simulink model "LIM_MO_Pso"  (R2016a)
settings: Solver=ode45  StartTime=0.0  StopTime=5
InitFcn:
  | %LIM in d-q referance
  | 
  |       Rs = 1.25;
  |       Rr = 2.7;
  |       Ls = 40.1e-3;
  |       Lr = 33.1e-3;
  |       Lm = 32.6e-3;
  |       tau =  0.0641;
  |       p = 4;
  |       D = 0.286;
  |       m = 8;
  |       ff=0;
  |      Tr=Lr/Rr;
  |     segma = 1-(Lm^2)/(Ls*Lr);
  |     sigma= segma;
  |        R=[Rs 0 0 0;0 Rs 0 0;0 0 Rr 0;0 0 0 Rr];
  |    R1=Rr*[1 0 1 0;0 0 0 0;1 0 1 0;0 0 0 0];%f(q)
  |    L=[Ls 0 0 0;0 Ls+Lm 0 Lm;0 0 Lr 0;0 Lm 0 Lr];
  |    L1=Lm*[1 0 1 0;0 0 0 0;1 0 1 0;0 0 0 0];%(1-f(q))
  |    M1=[0 -Ls-Lm 0 -Lm;Ls 0 0 0;0 0 0 0;0 0 0 0];
  |    M11=Lm*[0 0 0 0;1 0 1 0;0 0 0 0;0 0 0 0] ; %(1-f(q))
  |    M2=[0 0 0 0;0 0 0 0;0 -Lm 0 -Lr;0 0 Lr 0];
  |    M22=Lm*[0 0 0 0;0 0 0 0;0 0 0 0;1 0 1 0];%1-f(q)
  | 
  | 
  | Kpw = 7.8184
  | Kiw  = 55
  | Kpf = 6.9181
  | Kif = 996.637
  | Kpd = 8.9732
  | Kid  = 6792.1647
  | Kpq = 8.0997
  | Kiq = 6387.3475
StopFcn:
  |  figure(1)
  | plot(t,w,'LineWidth',2)
  | xlabel ('Time (s)','FontWeight','bold','FontSize',12)
  | ylabel ('speed (m/s)','FontWeight','bold','FontSize',12)
  | grid
  | 
  | 
  | figure(2)
  | plot(t,FF,'LineWidth',2)
  | xlabel ('Time (s)','FontWeight','bold','FontSize',12)
  | ylabel ('Thrust force (N)','FontWeight','bold','FontSize',12)
  | grid
  | 
  | 
  | figure(3)
  | plot(t,ids,'LineWidth',2)
  | xlabel ('Time (s)','FontWeight','bold','FontSize',12)
  | ylabel ('ids (A)','FontWeight','bold','FontSize',12)
  | grid
  | 
  | 
  | figure(4)
  | plot(t,iqs,'LineWidth',2)
  | xlabel ('Time (s)','FontWeight','bold','FontSize',12)
  | ylabel ('iqs (A)','FontWeight','bold','FontSize',12)
  | grid
  | 
  | figure(5)
  | plot(t,phdr,'LineWidth',2)
  | xlabel ('Time (s)','FontWeight','bold','FontSize',12)
  | ylabel ('phdr (Wb)','FontWeight','bold','FontSize',12)
  | grid
  | 
  | figure(6)
  | plot(t,phqr,'LineWidth',2)
  | xlabel ('Time (s)','FontWeight','bold','FontSize',12)
  | ylabel ('phqr (Wb)','FontWeight','bold','FontSize',12)
  | grid
libraries: simulink_need_slupdate x2, simulink x2
settings Model: Creator=DaLLaL  LastModifiedBy=DaLLaL
settings DebuggingCC: MaxConsecutiveZCsMsg=none

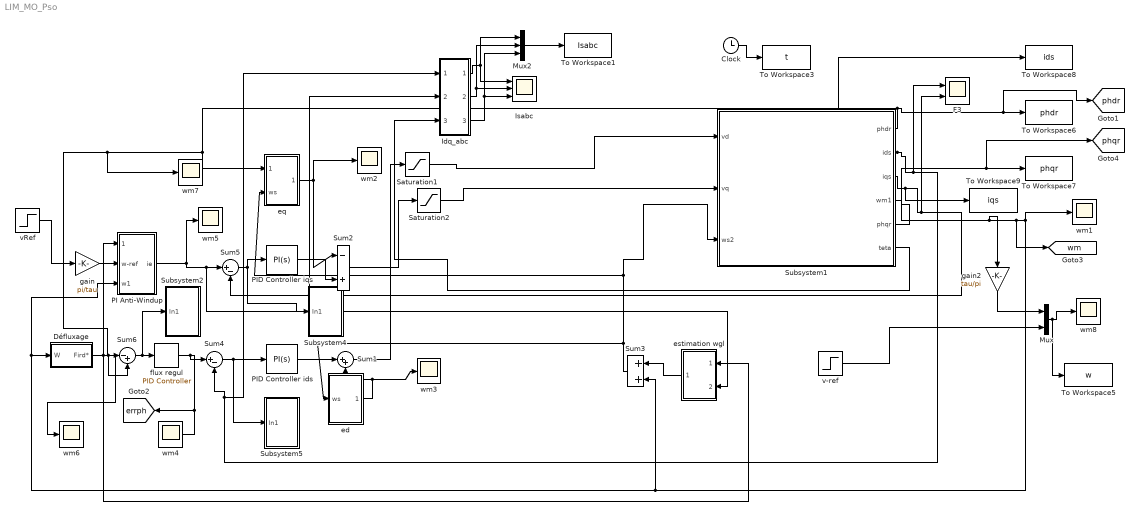
== system LIM_MO_Pso ==
  Clock : Clock
  Défluxage : Subsystem  mask{fref=0.4, Wn=300}
      mask prompts: fref "flux reference"; Wn "vitesse nominale"
  F3 : Scope  NumInputPorts=2
  Idq_abc : Subsystem
  Isabc : Scope  NumInputPorts=3
  Mux : Mux  Inputs=2
  Mux2 : Mux  Inputs=3
  PI Anti-Windup : Subsystem
  PID Controller ids : simulink/Continuous/PID Controller  Controller=PI  TimeDomain=Continuous-time  SampleTime=-1  IntegratorMethod=Forward Euler  FilterMethod=Forward Euler  Form=Parallel  UseFilter=on  ControllerParametersSource=internal  P=Kpd  I=Kid  D=0  N=100  InitialConditionSource=internal  InitialConditionForIntegrator=0  InitialConditionForFilter=0  ExternalReset=none  LimitOutput=off  UpperSaturationLimit=inf  LowerSaturationLimit=-inf  LinearizeAsGain=off  AntiWindupMode=none  Kb=1  TrackingMode=off  Kt=1  PParamMin=[]  PParamMax=[]  IParamMin=[]  IParamMax=[]  DParamMin=[]  DParamMax=[]  NParamMin=[]  NParamMax=[]  KbParamMin=[]  KbParamMax=[]  KtParamMin=[]  KtParamMax=[]  POutMin=[]  POutMax=[]  IOutMin=[]  IOutMax=[]  DOutMin=[]  DOutMax=[]  NOutMin=[]  NOutMax=[]  KbOutMin=[]  KbOutMax=[]  KtOutMin=[]  KtOutMax=[]  IntegratorOutMin=[]  IntegratorOutMax=[]  FilterOutMin=[]  FilterOutMax=[]  SumOutMin=[]  SumOutMax=[]  SumI1OutMin=[]  SumI1OutMax=[]  SumI2OutMin=[]  SumI2OutMax=[]  SumI3OutMin=[]  SumI3OutMax=[]  SumDOutMin=[]  SumDOutMax=[]  SaturationOutMin=[]  SaturationOutMax=[]  IntegratorContinuousStateAttributes=''  IntegratorStateMustResolveToSignalObject=off  IntegratorRTWStateStorageClass=Auto  FilterContinuousStateAttributes=''  FilterStateMustResolveToSignalObject=off  FilterRTWStateStorageClass=Auto  DifferentiatorICPrevScaledInput=0  DifferentiatorOutMin=[]  DifferentiatorOutMax=[]
  PID Controller iqs : simulink/Continuous/PID Controller  Controller=PI  TimeDomain=Continuous-time  SampleTime=-1  IntegratorMethod=Forward Euler  FilterMethod=Forward Euler  Form=Parallel  UseFilter=on  ControllerParametersSource=internal  P=Kpq  I=Kiq  D=0  N=100  InitialConditionSource=internal  InitialConditionForIntegrator=0  InitialConditionForFilter=0  ExternalReset=none  LimitOutput=off  UpperSaturationLimit=inf  LowerSaturationLimit=-inf  LinearizeAsGain=off  AntiWindupMode=none  Kb=1  TrackingMode=off  Kt=1  PParamMin=[]  PParamMax=[]  IParamMin=[]  IParamMax=[]  DParamMin=[]  DParamMax=[]  NParamMin=[]  NParamMax=[]  KbParamMin=[]  KbParamMax=[]  KtParamMin=[]  KtParamMax=[]  POutMin=[]  POutMax=[]  IOutMin=[]  IOutMax=[]  DOutMin=[]  DOutMax=[]  NOutMin=[]  NOutMax=[]  KbOutMin=[]  KbOutMax=[]  KtOutMin=[]  KtOutMax=[]  IntegratorOutMin=[]  IntegratorOutMax=[]  FilterOutMin=[]  FilterOutMax=[]  SumOutMin=[]  SumOutMax=[]  SumI1OutMin=[]  SumI1OutMax=[]  SumI2OutMin=[]  SumI2OutMax=[]  SumI3OutMin=[]  SumI3OutMax=[]  SumDOutMin=[]  SumDOutMax=[]  SaturationOutMin=[]  SaturationOutMax=[]  IntegratorContinuousStateAttributes=''  IntegratorStateMustResolveToSignalObject=off  IntegratorRTWStateStorageClass=Auto  FilterContinuousStateAttributes=''  FilterStateMustResolveToSignalObject=off  FilterRTWStateStorageClass=Auto  DifferentiatorICPrevScaledInput=0  DifferentiatorOutMin=[]  DifferentiatorOutMax=[]
  Saturation1 : Saturate  UpperLimit=600  LowerLimit=-600
  Saturation2 : Saturate  UpperLimit=600  LowerLimit=-600
  Subsystem1 : Subsystem
  Subsystem2 : Subsystem
  Subsystem4 : Subsystem
  Subsystem5 : Subsystem
  Sum1 : Sum  Inputs=|++
  Sum2 : Sum  Inputs=|-+
  Sum3 : Sum  Inputs=|++
  Sum4 : Sum  Inputs=|+-
  Sum5 : Sum  Inputs=|+-
  Sum6 : Sum  Inputs=|-+
  To Workspace1 : ToWorkspace  VariableName=Isabc  SampleTime=-1
  To Workspace3 : ToWorkspace  VariableName=t  SampleTime=-1
  To Workspace5 : ToWorkspace  VariableName=w  SampleTime=-1
  To Workspace6 : ToWorkspace  VariableName=phdr  SampleTime=-1
  To Workspace7 : ToWorkspace  VariableName=phqr  SampleTime=-1
  To Workspace8 : ToWorkspace  VariableName=ids  SampleTime=-1
  To Workspace9 : ToWorkspace  VariableName=iqs  SampleTime=-1
  ed : Subsystem
  eq : Subsystem
  estimation wgl : Subsystem
  flux regul : simulink_need_slupdate/PID Controller  P=Kpf  I=Kif  D=0
  gain : Gain  Gain=pi/tau
  gain2 : Gain  Gain=tau/pi
  v-ref : Step  Time=4  Before=3  After=4  SampleTime=0
  vRef : Step  Time=4  Before=3  After=4  SampleTime=0
  wm{1..8} (8 alike) : Scope
  tag scope: errph=global, phdr=global, phqr=global, wm=global
  wires:
  Subsystem1/2(ids) -> F3/1, Idq_abc/1(Vd), Sum4/2, To Workspace8/1
  Sum4/1 -> Subsystem5/1(In1), PID Controller ids/1
  Subsystem1/3(iqs) -> F3/2, Sum5/2, Idq_abc/2(Vq), To Workspace9/1
  Subsystem1/1(phdr) -> [phdr], To Workspace6/1, eq/1(phdr), Sum6/1, wm7/1
  PID Controller ids/1 -> Sum1/1
  eq/1(eqs) -> Sum2/1, wm2/1
  PI Anti-Windup/1(ie) -> Sum5/1, estimation wgl/2(iqsref), wm5/1
  Sum5/1 -> Subsystem4/1(In1), PID Controller iqs/1
  flux regul/1 -> Sum4/1, wm4/1, [errph]
  Défluxage/1(Fird*) -> wm6/1, Sum6/2, estimation wgl/1(phdr), PI Anti-Windup/1(phder)
  Sum3/1 -> Subsystem1/3(ws2), eq/2(ws), ed/1(ws)
  PID Controller iqs/1 -> Sum2/2
  Sum6/1 -> Subsystem2/1(In1), flux regul/1
  Subsystem1/5(phqr) -> [phqr], To Workspace7/1
  Mux/1 -> wm8/1, To Workspace5/1
  estimation wgl/1(wgl) -> Sum3/1
  Subsystem1/4(wm1) -> gain2/1, [wm], wm1/1, PI Anti-Windup/3(w1), Défluxage/1(W), Sum3/2
  Clock/1 -> To Workspace3/1
  ed/1(eds) -> Sum1/2, wm3/1
  Subsystem1/6(teta) -> Idq_abc/3(teta)
  Sum2/1 -> Saturation2/1
  Sum1/1 -> Saturation1/1
  vRef/1 -> gain/1
  gain/1 -> PI Anti-Windup/2(w-ref)
  v-ref/1 -> Mux/2
  Idq_abc/3(Vc) -> Mux2/3, Isabc/3
  Idq_abc/2(Vb) -> Mux2/2, Isabc/2
  Idq_abc/1(Va) -> Mux2/1, Isabc/1
  Mux2/1 -> To Workspace1/1
  gain2/1 -> Mux/1
  Saturation1/1 -> Subsystem1/1(vd)
  Saturation2/1 -> Subsystem1/2(vq)

== system LIM_MO_Pso/Défluxage ==
  W : Inport
  defluxage : Subsystem  mask(Defluxage){Phiref=1, Wn=Wn}
      mask prompts: Phiref "Phiref :"; Wn "Wn :"
      mask help: Defluxage
  Fird* : Outport
  wires:
  defluxage/1(fref) -> Fird*/1
  W/1 -> defluxage/1(w)

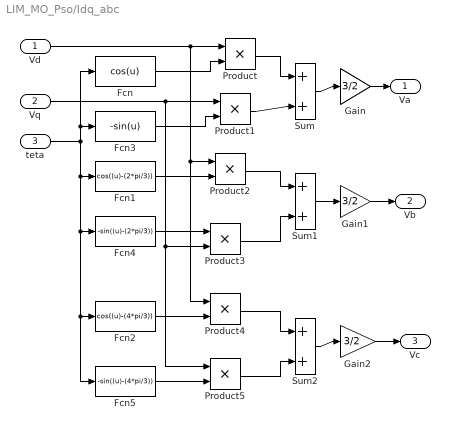
== system LIM_MO_Pso/Idq_abc ==
  Vd : Inport
  Vq : Inport  Port=2
  teta : Inport  Port=3
  Fcn : Fcn  Expr=cos(u)
  Fcn1 : Fcn  Expr=cos((u)-(2*pi/3))
  Fcn2 : Fcn  Expr=cos((u)-(4*pi/3))
  Fcn3 : Fcn  Expr=-sin(u)
  Fcn4 : Fcn  Expr=-sin((u)-(2*pi/3))
  Fcn5 : Fcn  Expr=-sin((u)-(4*pi/3))
  Gain : Gain  Gain=3/2  SaturateOnIntegerOverflow=on  OutDataTypeStr=Inherit: Same as input  ParamDataTypeStr=Inherit: Same as input
  Gain1 : Gain  Gain=3/2  SaturateOnIntegerOverflow=on  OutDataTypeStr=Inherit: Same as input  ParamDataTypeStr=Inherit: Same as input
  Gain2 : Gain  Gain=3/2  SaturateOnIntegerOverflow=on  OutDataTypeStr=Inherit: Same as input  ParamDataTypeStr=Inherit: Same as input
  Product{,1..5} (6 alike) : Product  SaturateOnIntegerOverflow=on  InputSameDT=on  OutDataTypeStr=Inherit: Same as first input
  Sum : Sum  Inputs=|++  SaturateOnIntegerOverflow=on  InputSameDT=on  OutDataTypeStr=Inherit: Same as first input
  Sum1 : Sum  Inputs=|++  SaturateOnIntegerOverflow=on  InputSameDT=on  OutDataTypeStr=Inherit: Same as first input
  Sum2 : Sum  Inputs=|++  SaturateOnIntegerOverflow=on  InputSameDT=on  OutDataTypeStr=Inherit: Same as first input
  Va : Outport
  Vb : Outport  Port=2
  Vc : Outport  Port=3
  wires:
  Gain2/1 -> Vc/1
  Gain1/1 -> Vb/1
  Gain/1 -> Va/1
  Sum2/1 -> Gain2/1
  Sum1/1 -> Gain1/1
  Sum/1 -> Gain/1
  Product5/1 -> Sum2/2
  Product4/1 -> Sum2/1
  Product3/1 -> Sum1/2
  Product2/1 -> Sum1/1
  Product1/1 -> Sum/2
  Product/1 -> Sum/1
  teta/1 -> Fcn5/1, Fcn2/1, Fcn4/1, Fcn1/1, Fcn3/1, Fcn/1
  Fcn5/1 -> Product5/2
  Fcn2/1 -> Product4/2
  Fcn4/1 -> Product3/1
  Fcn1/1 -> Product2/2
  Vq/1 -> Product5/1, Product3/2, Product1/1
  Vd/1 -> Product4/1, Product2/1, Product/1
  Fcn3/1 -> Product1/2
  Fcn/1 -> Product/2

== system LIM_MO_Pso/PI Anti-Windup ==
  phder : Inport
  w-ref : Inport  Port=2
  w1 : Inport  Port=3
  PID Controller2 : simulink_need_slupdate/PID Controller  P=Kpw  I=Kiw  D=0
  Subsystem : Subsystem
  Subsystem2 : Subsystem
  Sum : Sum  Inputs=|+-  SaturateOnIntegerOverflow=on
  ie : Outport
  wires:
  Sum/1 -> PID Controller2/1
  PID Controller2/1 -> Subsystem2/1(In1), Subsystem/2(ce*)
  phder/1 -> Subsystem/1(phder)
  w1/1 -> Sum/2
  w-ref/1 -> Sum/1
  Subsystem/1(ie*) -> ie/1

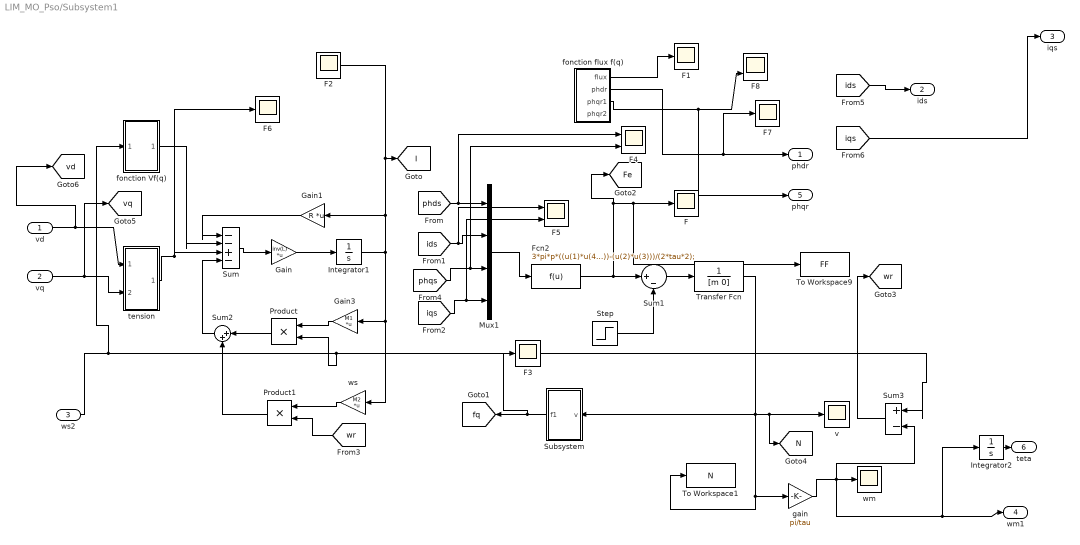
== system LIM_MO_Pso/Subsystem1 ==
  vd : Inport
  vq : Inport  Port=2
  ws2 : Inport  Port=3
  F{,1..3,6..7} (6 alike) : Scope
  F4 : Scope  NumInputPorts=2
  F5 : Scope  NumInputPorts=2
  F8 : Scope  NumInputPorts=2
  Fcn2 : Fcn  Expr=3*pi*p*((u(1)*u(4))-(u(2)*u(3)))/(2*tau*2);
  Gain : Gain  Gain=inv(L)  Multiplication=Matrix(K*u)
  Gain1 : Gain  Gain=R  Multiplication=Matrix(K*u)
  Gain3 : Gain  Gain=M1  Multiplication=Matrix(K*u)
  Integrator1 : Integrator
  Integrator2 : Integrator
  Mux1 : Mux
  Product : Product  RndMeth=Zero
  Product1 : Product  RndMeth=Zero
  Step : Step  After=50  SampleTime=0
  Subsystem : Subsystem
  Sum : Sum  Inputs=|--+-
  Sum1 : Sum  Inputs=|+-
  Sum2 : Sum  Inputs=|++
  Sum3 : Sum  Inputs=|+-
  To Workspace1 : ToWorkspace  VariableName=N  SampleTime=-1
  To Workspace9 : ToWorkspace  VariableName=FF  SampleTime=-1
  Transfer Fcn : TransferFcn  Denominator=[m 0]
  fonction Vf(q) : Subsystem
  fonction flux f(q) : Subsystem
  gain : Gain  Gain=pi/tau
  tension : Subsystem
  v : Scope
  wm : Scope
  ws : Gain  Gain=M2  Multiplication=Matrix(K*u)
  phdr : Outport
  ids : Outport  Port=2
  iqs : Outport  Port=3
  wm1 : Outport  Port=4
  phqr : Outport  Port=5
  teta : Outport  Port=6
  tag scope: Fe=global, I=global, N=global, fq=global, vd=global, vq=global, wr=global
  wires:
  Gain/1 -> Integrator1/1
  Integrator1/1 -> Gain3/1, ws/1, Gain1/1, [I], F2/1
  Gain3/1 -> Product/1
  Sum/1 -> Gain/1
  ws/1 -> Product1/1
  Product1/1 -> Sum2/2
  Product/1 -> Sum2/1
  [wr] -> Product1/2
  Gain1/1 -> Sum/1
  Sum2/1 -> Sum/4
  Subsystem/1(f1) -> [fq], F3/1
  fonction Vf(q)/1(Out1) -> Sum/2
  Fcn2/1 -> [Fe], F/1, To Workspace9/1, Sum1/1
  Step/1 -> Sum1/2
  Sum1/1 -> Transfer Fcn/1
  Transfer Fcn/1 -> To Workspace1/1, gain/1, [N], v/1, Subsystem/1(v)
  gain/1 -> wm/1, Sum3/2, wm1/1, Integrator2/1
  Sum3/1 -> [wr]
  [phds] -> Mux1/1, F4/1
  [ids] -> Mux1/2, F5/1
  [iqs] -> Mux1/4, F5/2
  [phqs] -> Mux1/3, F4/2
  Mux1/1 -> Fcn2/1
  fonction flux f(q)/1(flux) -> F1/1
  fonction flux f(q)/2(phdr) -> phdr/1, F7/1
  [ids] -> ids/1
  [iqs] -> iqs/1
  tension/1(V (v)) -> Sum/3, F6/1
  ws2/1 -> Product/2, Sum3/1, fonction Vf(q)/1(ws2)
  vd/1 -> [vd], tension/1(In2)
  vq/1 -> [vq], tension/2(In1)
  fonction flux f(q)/3(phqr1) -> F8/2, phqr/1
  Integrator2/1 -> teta/1

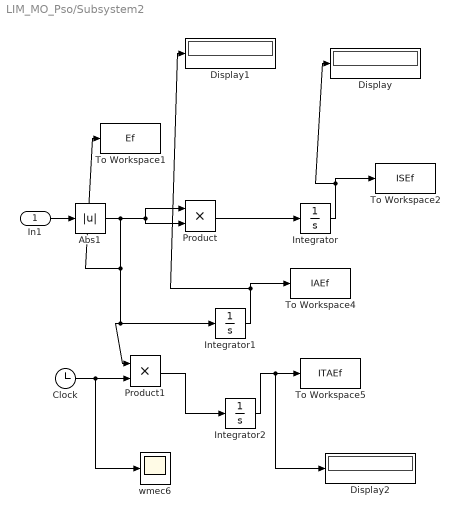
== system LIM_MO_Pso/Subsystem2 ==
  In1 : Inport
  Abs1 : Abs
  Clock : Clock
      settings: Decimation=4
  Display : Display
  Display1 : Display
  Display2 : Display
  Integrator : Integrator
  Integrator1 : Integrator
  Integrator2 : Integrator
  Product : Product  RndMeth=Zero
  Product1 : Product  RndMeth=Zero
  To Workspace1 : ToWorkspace  VariableName=Ef  SampleTime=-1
      settings: MaxDataPoints=1
  To Workspace2 : ToWorkspace  VariableName=ISEf  SampleTime=-1
      settings: MaxDataPoints=1
  To Workspace4 : ToWorkspace  VariableName=IAEf  SampleTime=-1
      settings: MaxDataPoints=1
  To Workspace5 : ToWorkspace  VariableName=ITAEf  SampleTime=-1
      settings: MaxDataPoints=1
  wmec6 : Scope
  wires:
  In1/1 -> Abs1/1
  Product1/1 -> Integrator2/1
  Integrator2/1 -> Display2/1, To Workspace5/1
  Clock/1 -> Product1/2, wmec6/1
  Integrator1/1 -> Display1/1, To Workspace4/1
  Abs1/1 -> Product/1, Product/2, Product1/1, Integrator1/1, To Workspace1/1
  Integrator/1 -> Display/1, To Workspace2/1
  Product/1 -> Integrator/1

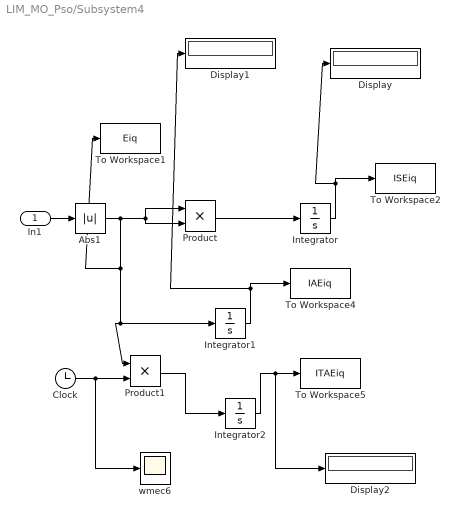
== system LIM_MO_Pso/Subsystem4 ==
  In1 : Inport
  Abs1 : Abs
  Clock : Clock
      settings: Decimation=4
  Display : Display
  Display1 : Display
  Display2 : Display
  Integrator : Integrator
  Integrator1 : Integrator
  Integrator2 : Integrator
  Product : Product  RndMeth=Zero
  Product1 : Product  RndMeth=Zero
  To Workspace1 : ToWorkspace  VariableName=Eiq  SampleTime=-1
      settings: MaxDataPoints=1
  To Workspace2 : ToWorkspace  VariableName=ISEiq  SampleTime=-1
      settings: MaxDataPoints=1
  To Workspace4 : ToWorkspace  VariableName=IAEiq  SampleTime=-1
      settings: MaxDataPoints=1
  To Workspace5 : ToWorkspace  VariableName=ITAEiq  SampleTime=-1
      settings: MaxDataPoints=1
  wmec6 : Scope
  wires:
  Product/1 -> Integrator/1
  Integrator/1 -> To Workspace2/1, Display/1
  Abs1/1 -> To Workspace1/1, Integrator1/1, Product1/1, Product/2, Product/1
  Integrator1/1 -> To Workspace4/1, Display1/1
  Clock/1 -> wmec6/1, Product1/2
  Integrator2/1 -> To Workspace5/1, Display2/1
  Product1/1 -> Integrator2/1
  In1/1 -> Abs1/1

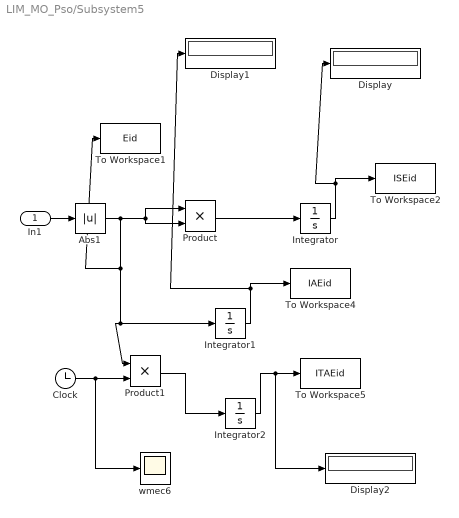
== system LIM_MO_Pso/Subsystem5 ==
  In1 : Inport
  Abs1 : Abs
  Clock : Clock
      settings: Decimation=4
  Display : Display
  Display1 : Display
  Display2 : Display
  Integrator : Integrator
  Integrator1 : Integrator
  Integrator2 : Integrator
  Product : Product  RndMeth=Zero
  Product1 : Product  RndMeth=Zero
  To Workspace1 : ToWorkspace  VariableName=Eid  SampleTime=-1
      settings: MaxDataPoints=1
  To Workspace2 : ToWorkspace  VariableName=ISEid  SampleTime=-1
      settings: MaxDataPoints=1
  To Workspace4 : ToWorkspace  VariableName=IAEid  SampleTime=-1
      settings: MaxDataPoints=1
  To Workspace5 : ToWorkspace  VariableName=ITAEid  SampleTime=-1
      settings: MaxDataPoints=1
  wmec6 : Scope
  wires:
  In1/1 -> Abs1/1
  Product1/1 -> Integrator2/1
  Integrator2/1 -> Display2/1, To Workspace5/1
  Clock/1 -> Product1/2, wmec6/1
  Integrator1/1 -> Display1/1, To Workspace4/1
  Abs1/1 -> Product/1, Product/2, Product1/1, Integrator1/1, To Workspace1/1
  Integrator/1 -> Display/1, To Workspace2/1
  Product/1 -> Integrator/1

== system LIM_MO_Pso/ed ==
  ws : Inport
  Gain2 : Gain  Gain=(Ls+Lm)-(Lm*Lm/(Lm+Lr))
  Product2 : Product  RndMeth=Zero
  eds : Outport
  wires:
  ws/1 -> Gain2/1
  [iqs] -> Product2/1
  Gain2/1 -> Product2/2
  Product2/1 -> eds/1

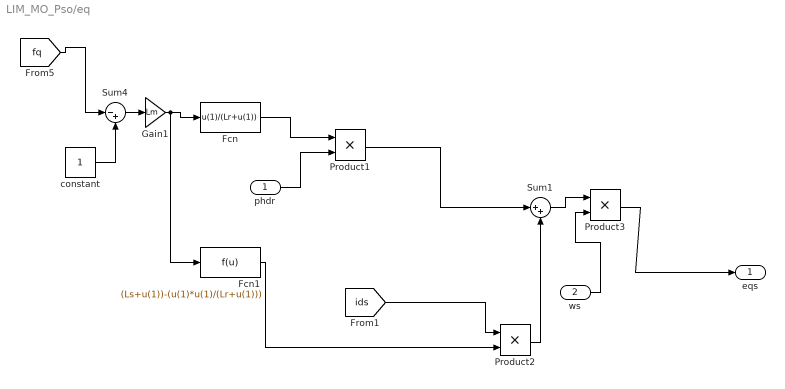
== system LIM_MO_Pso/eq ==
  phdr : Inport
  ws : Inport  Port=2
  Fcn : Fcn  Expr=u(1)/(Lr+u(1))
  Fcn1 : Fcn  Expr=(Ls+u(1))-(u(1)*u(1)/(Lr+u(1)))
  Gain1 : Gain  Gain=Lm
  Product1 : Product  RndMeth=Zero
  Product2 : Product  RndMeth=Zero
  Product3 : Product  RndMeth=Zero
  Sum1 : Sum  Inputs=|++
  Sum4 : Sum  Inputs=|-+
  constant : Constant
  eqs : Outport
  wires:
  [fq] -> Sum4/1
  constant/1 -> Sum4/2
  Sum4/1 -> Gain1/1
  [ids] -> Product2/1
  Fcn1/1 -> Product2/2
  phdr/1 -> Product1/2
  Fcn/1 -> Product1/1
  Gain1/1 -> Fcn/1, Fcn1/1
  Product1/1 -> Sum1/1
  Product2/1 -> Sum1/2
  Sum1/1 -> Product3/1
  ws/1 -> Product3/2
  Product3/1 -> eqs/1

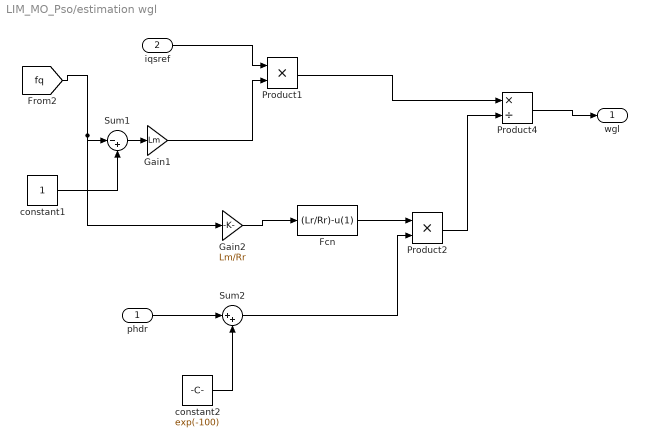
== system LIM_MO_Pso/estimation wgl ==
  phdr : Inport
  iqsref : Inport  Port=2
  Fcn : Fcn  Expr=(Lr/Rr)-u(1)
  Gain1 : Gain  Gain=Lm
  Gain2 : Gain  Gain=Lm/Rr
  Product1 : Product  RndMeth=Zero
  Product2 : Product  RndMeth=Zero
  Product4 : Product  Inputs=*/  RndMeth=Zero
  Sum1 : Sum  Inputs=|-+
  Sum2 : Sum  Inputs=|++
  constant1 : Constant
  constant2 : Constant  Value=exp(-100)
  wgl : Outport
  wires:
  phdr/1 -> Sum2/1
  constant2/1 -> Sum2/2
  iqsref/1 -> Product1/1
  Product4/1 -> wgl/1
  [fq] -> Sum1/1, Gain2/1
  constant1/1 -> Sum1/2
  Sum1/1 -> Gain1/1
  Gain1/1 -> Product1/2
  Gain2/1 -> Fcn/1
  Fcn/1 -> Product2/1
  Sum2/1 -> Product2/2
  Product2/1 -> Product4/2
  Product1/1 -> Product4/1

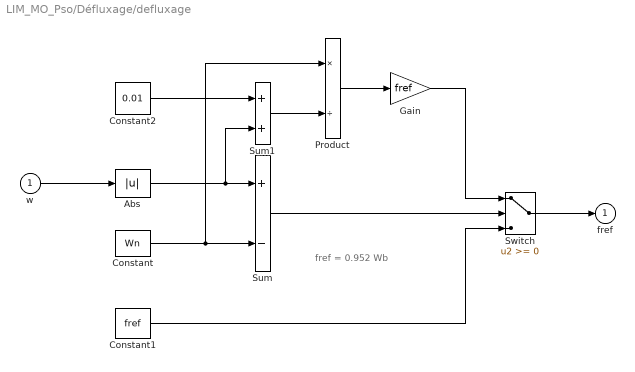
== system LIM_MO_Pso/Défluxage/defluxage ==
  note: fref = 0.952 Wb
  w : Inport
  Abs : Abs  SaturateOnIntegerOverflow=on
  Constant : Constant  Value=Wn
  Constant1 : Constant  Value=fref
  Constant2 : Constant  Value=0.01
  Gain : Gain  Gain=fref  SaturateOnIntegerOverflow=on  OutDataTypeStr=Inherit: Same as input  ParamDataTypeStr=Inherit: Same as input
  Product : Product  Inputs=*/  SaturateOnIntegerOverflow=on  OutDataTypeStr=Inherit: Same as first input
  Sum : Sum  Inputs=+-  SaturateOnIntegerOverflow=on  InputSameDT=on  OutDataTypeStr=Inherit: Same as first input
  Sum1 : Sum  SaturateOnIntegerOverflow=on  InputSameDT=on  OutDataTypeStr=Inherit: Same as first input
  Switch : Switch  SaturateOnIntegerOverflow=on  InputSameDT=on
  fref : Outport  InitialOutput=0
  wires:
  Sum1/1 -> Product/2
  Constant2/1 -> Sum1/1
  Switch/1 -> fref/1
  w/1 -> Abs/1
  Sum/1 -> Switch/2
  Constant/1 -> Product/1, Sum/2
  Abs/1 -> Sum1/2, Sum/1
  Product/1 -> Gain/1
  Gain/1 -> Switch/1
  Constant1/1 -> Switch/3

== system LIM_MO_Pso/PI Anti-Windup/Subsystem ==
  phder : Inport
  ce* : Inport  Port=2
  Subsystem : Subsystem
  ie* : Outport
  wires:
  Subsystem/1(ie*) -> ie*/1
  phder/1 -> Subsystem/2(phder)
  ce*/1 -> Subsystem/1(In2)

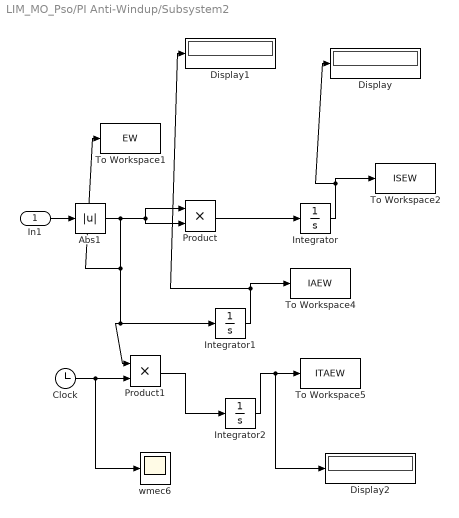
== system LIM_MO_Pso/PI Anti-Windup/Subsystem2 ==
  In1 : Inport
  Abs1 : Abs
  Clock : Clock
      settings: Decimation=4
  Display : Display
  Display1 : Display
  Display2 : Display
  Integrator : Integrator
  Integrator1 : Integrator
  Integrator2 : Integrator
  Product : Product  RndMeth=Zero
  Product1 : Product  RndMeth=Zero
  To Workspace1 : ToWorkspace  VariableName=EW  SampleTime=-1
      settings: MaxDataPoints=1
  To Workspace2 : ToWorkspace  VariableName=ISEW  SampleTime=-1
      settings: MaxDataPoints=1
  To Workspace4 : ToWorkspace  VariableName=IAEW  SampleTime=-1
      settings: MaxDataPoints=1
  To Workspace5 : ToWorkspace  VariableName=ITAEW  SampleTime=-1
      settings: MaxDataPoints=1
  wmec6 : Scope
  wires:
  In1/1 -> Abs1/1
  Product1/1 -> Integrator2/1
  Integrator2/1 -> Display2/1, To Workspace5/1
  Clock/1 -> Product1/2, wmec6/1
  Integrator1/1 -> Display1/1, To Workspace4/1
  Abs1/1 -> Product/1, Product/2, Product1/1, Integrator1/1, To Workspace1/1
  Integrator/1 -> Display/1, To Workspace2/1
  Product/1 -> Integrator/1

== system LIM_MO_Pso/Subsystem1/Subsystem ==
  v : Inport
  Q : Fcn  Expr=abs(D*Rr/(Lr*u(1)))
  f : Fcn  Expr=(1-exp(-u(1)))/u(1)
  f1 : Outport
  wires:
  Q/1 -> f/1
  f/1 -> f1/1
  v/1 -> Q/1

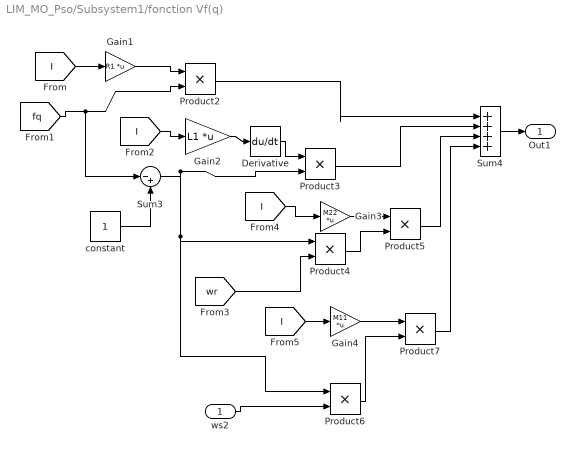
== system LIM_MO_Pso/Subsystem1/fonction Vf(q) ==
  ws2 : Inport
  Derivative : Derivative
  Gain1 : Gain  Gain=R1  Multiplication=Matrix(K*u)
  Gain2 : Gain  Gain=L1  Multiplication=Matrix(K*u)
  Gain3 : Gain  Gain=M22  Multiplication=Matrix(K*u)
  Gain4 : Gain  Gain=M11  Multiplication=Matrix(K*u)
  Product{2..7} (6 alike) : Product  RndMeth=Zero
  Sum3 : Sum  Inputs=|-+
  Sum4 : Sum  Inputs=|++++
  constant : Constant
  Out1 : Outport
  wires:
  [fq] -> Sum3/1, Product2/2
  [I] -> Gain1/1
  constant/1 -> Sum3/2
  Sum3/1 -> Product4/1, Product6/1, Product3/2
  [I] -> Gain2/1
  [wr] -> Product4/2
  Product4/1 -> Product5/2
  ws2/1 -> Product6/2
  Product6/1 -> Product7/2
  [I] -> Gain4/1
  Product7/1 -> Sum4/4
  Product5/1 -> Sum4/3
  Product3/1 -> Sum4/2
  Product2/1 -> Sum4/1
  Derivative/1 -> Product3/1
  Sum4/1 -> Out1/1
  Gain1/1 -> Product2/1
  Gain2/1 -> Derivative/1
  [I] -> Gain3/1
  Gain3/1 -> Product5/1
  Gain4/1 -> Product7/1

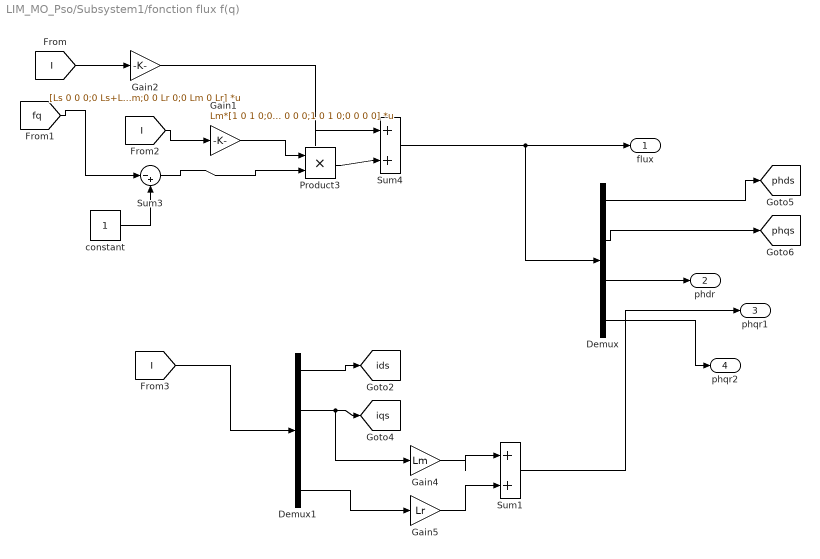
== system LIM_MO_Pso/Subsystem1/fonction flux f(q) ==
  Demux : Demux
  Demux1 : Demux
  Gain1 : Gain  Gain=Lm*[1 0 1 0;0 0 0 0;1 0 1 0;0 0 0 0]  Multiplication=Matrix(K*u)
  Gain2 : Gain  Gain=[Ls 0 0 0;0 Ls+Lm 0 Lm;0 0 Lr 0;0 Lm 0 Lr]  Multiplication=Matrix(K*u)
  Gain4 : Gain  Gain=Lm
  Gain5 : Gain  Gain=Lr
  Product3 : Product  RndMeth=Zero
  Sum1 : Sum  Inputs=|++
  Sum3 : Sum  Inputs=|-+
  Sum4 : Sum  Inputs=|++
  constant : Constant
  flux : Outport
  phdr : Outport  Port=2
  phqr1 : Outport  Port=3
  phqr2 : Outport  Port=4
  tag scope: ids=global, iqs=global, phds=global, phqs=global
  wires:
  Sum4/1 -> flux/1, Demux/1
  Product3/1 -> Sum4/2
  [I] -> Gain1/1
  Sum3/1 -> Product3/2
  constant/1 -> Sum3/2
  [fq] -> Sum3/1
  [I] -> Gain2/1
  Gain2/1 -> Sum4/1
  [I] -> Demux1/1
  Demux/1 -> [phds]
  Demux/2 -> [phqs]
  Demux1/1 -> [ids]
  Demux1/2 -> [iqs], Gain4/1
  Gain1/1 -> Product3/1
  Demux/3 -> phdr/1
  Demux1/4 -> Gain5/1
  Gain5/1 -> Sum1/2
  Gain4/1 -> Sum1/1
  Sum1/1 -> phqr1/1
  Demux/4 -> phqr2/1

== system LIM_MO_Pso/Subsystem1/tension ==
  In2 : Inport
  In1 : Inport  Port=2
  Mux1 : Mux
  Vdr;Vqr : Constant  Value=0
  V (v) : Outport
  wires:
  Vdr;Vqr/1 -> Mux1/3, Mux1/4
  Mux1/1 -> V (v)/1
  In2/1 -> Mux1/1
  In1/1 -> Mux1/2

== system LIM_MO_Pso/PI Anti-Windup/Subsystem/Subsystem ==
  In2 : Inport
  phder : Inport  Port=2
  Constant : Constant  Value=exp(-100)
  Divide : Product  Inputs=*/
  Gain : Gain  Gain=((Lr+Lm)/Lm)*(4*tau)/(3*pi*p)
  Sum1 : Sum  Inputs=|++  SaturateOnIntegerOverflow=on
  ie* : Outport
  wires:
  Divide/1 -> Gain/1
  phder/1 -> Sum1/1
  Sum1/1 -> Divide/2
  Constant/1 -> Sum1/2
  Gain/1 -> ie*/1
  In2/1 -> Divide/1
